simulink model "three"  (R2014b)
settings: Solver=ode23tb  StartTime=0.0  StopTime=0.1  MaxStep=.0001  MinStep=0.00001  RelTol=1e-3
libraries: powerlib x120, simulink x60, powerlib_meascontrol x1
(part 1 of 2)
settings Model: Creator=Muruganandham  LastModifiedBy=SELVA
settings DataIOCC: SignalLoggingSaveFormat=ModelDataLogs
settings OptimizationCC: ExpressionDepthLimit=2147483647
settings DebuggingCC: UnderspecifiedInitializationDetection=Classic  MergeDetectMultiDrivingBlocksExec=none  FcnCallInpInsideContextMsg=UseLocalSettings  StateNameClashWarn=warning
settings GRTTargetCC: CombineOutputUpdateFcns=off  GRTInterface=on

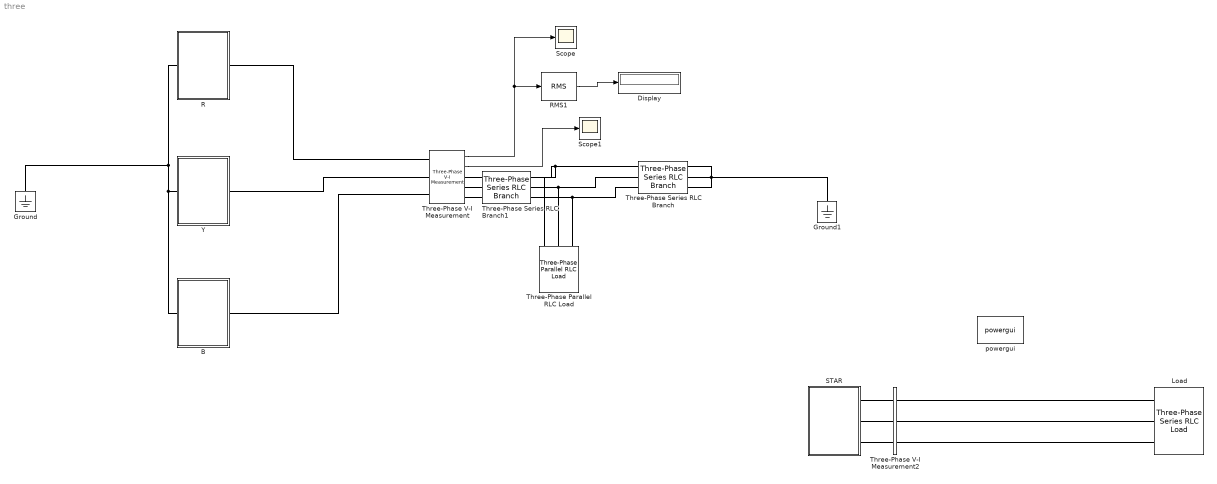
== system three ==
  " Load" : powerlib/Elements/Three-Phase Series RLC Load  LConnTagsString=A|B|C  Configuration=Delta  NominalVoltage=385  NominalFrequency=50  ActivePower=1000  InductivePower=0  CapacitivePower=0  Measurements=None  LoadType=constant Z
  "B " : Subsystem
  Display : Display
  Ground : powerlib/Elements/Ground  LConnTagsString=a
  Ground1 : powerlib/Elements/Ground  LConnTagsString=a
  R : Subsystem
  RMS1 : powerlib_meascontrol/Measurements/RMS  TrueRMS=on  Freq=50  RMSInit=00  Ts=0
  STAR : Subsystem
  Scope : Scope
      settings: YMin=-600  YMax=600  SaveName=bn  DataFormat=Structure
  Scope1 : Scope
      settings: YMin=-500  YMax=500  SaveName=ScopeData2
  Three-Phase Parallel RLC Load : powerlib/Elements/Three-Phase Parallel RLC Load  LConnTagsString=A|B|C  Configuration=Y (grounded)  NominalVoltage=380  NominalFrequency=50  ActivePower=00  InductivePower=000  CapacitivePower=3000  Measurements=None  LoadType=constant Z
  Three-Phase Series RLC Branch : powerlib/Elements/Three-Phase Series RLC Branch  LConnTagsString=A|B|C  RConnTagsString=A|B|C  BranchType=R  Resistance=10  Inductance=1e-3  Capacitance=1e-6  Measurements=None
  Three-Phase Series RLC Branch1 : powerlib/Elements/Three-Phase Series RLC Branch  LConnTagsString=A|B|C  RConnTagsString=A|B|C  BranchType=L  Resistance=10  Inductance=2e-3  Capacitance=1e-6  Measurements=None
  Three-Phase V-I Measurement : powerlib/Measurements/Three-Phase V-I Measurement  VoltageMeasurement=phase-to-phase  SetLabelV=off  LabelV=Vabc  Vpu=off  VpuLL=off  CurrentMeasurement=yes  SetLabelI=off  LabelI=Iabc  Ipu=off  Pbase=100e6  Vbase=500e3  OutputType=Complex  PhasorSimulation=off  PSBequivalent=0
  Three-Phase V-I Measurement2 : powerlib/Measurements/Three-Phase V-I Measurement  VoltageMeasurement=phase-to-phase  SetLabelV=on  LabelV=Vabc1  Vpu=off  VpuLL=off  CurrentMeasurement=yes  SetLabelI=on  LabelI=Iabc1  Ipu=off  Pbase=100e6  Vbase=500e3  OutputType=Complex  PhasorSimulation=off  PSBequivalent=0
  Y : Subsystem
  powergui : powerlib/powergui  Priority=1  SimulationMode=Discrete  SolverType=Tustin  SampleTime=50e-6  frequency=60  SPID=off  DisableSnubberDevices=off  DisableRonSwitches=off  DisableVfSwitches=off  SwTol=0  DisplayEquations=off  Interpol=off  methode=off  Ts=0  frequencyindice=0  Pbase=100e6  ErrMax=1e-4  Iterations=50  UnitsV=kV  UnitsW=MW  FunctionMessages=off  echomessages=off  HookPort=off  EnableUseOfTLC=off  x0status=blocks  RestoreLinks=warning  ResistiveCurrentMeasurement=off  Frange=[0:2:500]  Ylog=off  Xlog=on  ShowGrid=off  save=off  variable=ZData  structure=bn  ZoomFFT=off  StartTime=0.04  cycles=1  DisplayStyle=1  fundamental=50  FreqAxis=off  MaxFrequency=1000  frequencyindicesteady=1  RmsSteady=1  display=off
  wires:
  Three-Phase V-I Measurement/1 -> RMS1/1, Scope/1
  Three-Phase V-I Measurement/2 -> Scope1/1
  RMS1/1 -> Display/1
  connections:
  R/LConn1 -- Ground/LConn1 -- Y/LConn1 -- "B "/LConn1
  Three-Phase V-I Measurement/LConn1 -- R/RConn1
  Three-Phase V-I Measurement/LConn2 -- Y/RConn1
  Three-Phase V-I Measurement/LConn3 -- "B "/RConn1
  Three-Phase Series RLC Branch/LConn1 -- Three-Phase Series RLC Branch1/RConn1 -- Three-Phase Parallel RLC Load/LConn1
  Three-Phase Parallel RLC Load/LConn2 -- Three-Phase Series RLC Branch/LConn2 -- Three-Phase Series RLC Branch1/RConn2
  Three-Phase Series RLC Branch/LConn3 -- Three-Phase Parallel RLC Load/LConn3 -- Three-Phase Series RLC Branch1/RConn3
  Ground1/LConn1 -- Three-Phase Series RLC Branch/RConn3 -- Three-Phase Series RLC Branch/RConn1 -- Three-Phase Series RLC Branch/RConn2
  Three-Phase Series RLC Branch1/LConn1 -- Three-Phase V-I Measurement/RConn1
  Three-Phase V-I Measurement/RConn2 -- Three-Phase Series RLC Branch1/LConn2
  Three-Phase Series RLC Branch1/LConn3 -- Three-Phase V-I Measurement/RConn3
  STAR/LConn3 -- Three-Phase V-I Measurement2/LConn3
  Three-Phase V-I Measurement2/RConn2 -- " Load"/LConn2
  " Load"/LConn3 -- Three-Phase V-I Measurement2/RConn3
  Three-Phase V-I Measurement2/LConn2 -- STAR/LConn2
  Three-Phase V-I Measurement2/LConn1 -- STAR/LConn1
  Three-Phase V-I Measurement2/RConn1 -- " Load"/LConn1

== system three/B  ==
  B : Subsystem  mask{fc=10000, m=1}
      mask prompts: fc "Switching frequency"; m "modulation index"
  DC Voltage Source{1..3,5..6} (5 alike) : powerlib/Electrical Sources/DC Voltage Source  Amplitude=66.5  Measurements=None
  IGBT/Diode{,1..8,10..12} (12 alike) : powerlib/Power Electronics/IGBT//Diode  Ron=1e-3  Rs=1e5  Cs=inf  Measurements=on
  Scope : Scope
  Voltage Measurement : powerlib/Measurements/Voltage Measurement  PhasorSimulation=off  OutputType=Complex  PSBequivalent=0
  P : PMIOPort  Tag=PMCPort  Port=1  Side=Right
  N : PMIOPort  Tag=PMCPort  Port=2  Side=Left
  wires:
  [BS10] -> IGBT/Diode4/1
  [BS2] -> IGBT/Diode2/1
  [BS20] -> IGBT/Diode5/1
  [BS3] -> IGBT/Diode/1
  [BS30] -> IGBT/Diode3/1
  [BS40] -> IGBT/Diode8/1
  [BS6] -> IGBT/Diode6/1
  [BS4] -> IGBT/Diode12/1
  [BS5] -> IGBT/Diode7/1
  [BS50] -> IGBT/Diode10/1
  [BS60] -> IGBT/Diode11/1
  Voltage Measurement/1 -> Scope/1
  [BS1] -> IGBT/Diode1/1
  connections:
  IGBT/Diode2/RConn1 -- DC Voltage Source2/LConn1 -- IGBT/Diode/RConn1
  IGBT/Diode1/LConn1 -- DC Voltage Source1/RConn1 -- IGBT/Diode2/LConn1
  IGBT/Diode5/LConn1 -- DC Voltage Source2/RConn1 -- IGBT/Diode3/LConn1
  IGBT/Diode4/RConn1 -- DC Voltage Source1/LConn1 -- IGBT/Diode5/RConn1
  IGBT/Diode4/LConn1 -- IGBT/Diode1/RConn1 -- N/RConn1 -- Voltage Measurement/LConn2
  IGBT/Diode7/LConn1 -- DC Voltage Source6/RConn1 -- IGBT/Diode6/LConn1
  IGBT/Diode12/RConn1 -- DC Voltage Source3/LConn1 -- IGBT/Diode7/RConn1
  IGBT/Diode10/RConn1 -- DC Voltage Source6/LConn1 -- IGBT/Diode11/RConn1
  IGBT/Diode8/LConn1 -- DC Voltage Source3/RConn1 -- IGBT/Diode10/LConn1
  DC Voltage Source5/RConn1 -- IGBT/Diode/LConn1 -- IGBT/Diode12/LConn1
  DC Voltage Source5/LConn1 -- IGBT/Diode3/RConn1 -- IGBT/Diode8/RConn1
  IGBT/Diode6/RConn1 -- IGBT/Diode11/LConn1 -- P/RConn1 -- Voltage Measurement/LConn1

== system three/R ==
  DC Voltage Source{1..3,5..6} (5 alike) : powerlib/Electrical Sources/DC Voltage Source  Amplitude=66.5  Measurements=None
  IGBT/Diode{,1..8,10..12} (12 alike) : powerlib/Power Electronics/IGBT//Diode  Ron=1e-3  Rs=1e5  Cs=inf  Measurements=on
  R : Subsystem  mask{fc=10000, m=1}
      mask prompts: fc "Switching frequency"; m "modulation index"
  Scope : Scope
  Voltage Measurement : powerlib/Measurements/Voltage Measurement  PhasorSimulation=off  OutputType=Complex  PSBequivalent=0
  P : PMIOPort  Tag=PMCPort  Port=1  Side=Right
  N : PMIOPort  Tag=PMCPort  Port=2  Side=Left
  wires:
  [RS10] -> IGBT/Diode4/1
  [RS2] -> IGBT/Diode2/1
  [RS20] -> IGBT/Diode5/1
  [RS3] -> IGBT/Diode/1
  [RS30] -> IGBT/Diode3/1
  [RS40] -> IGBT/Diode8/1
  [RS6] -> IGBT/Diode6/1
  [RS4] -> IGBT/Diode12/1
  [RS5] -> IGBT/Diode7/1
  [RS50] -> IGBT/Diode10/1
  [RS60] -> IGBT/Diode11/1
  Voltage Measurement/1 -> Scope/1
  [RS1] -> IGBT/Diode1/1
  connections:
  IGBT/Diode2/RConn1 -- DC Voltage Source2/LConn1 -- IGBT/Diode/RConn1
  IGBT/Diode1/LConn1 -- DC Voltage Source1/RConn1 -- IGBT/Diode2/LConn1
  IGBT/Diode5/LConn1 -- DC Voltage Source2/RConn1 -- IGBT/Diode3/LConn1
  IGBT/Diode4/RConn1 -- DC Voltage Source1/LConn1 -- IGBT/Diode5/RConn1
  IGBT/Diode4/LConn1 -- Voltage Measurement/LConn2 -- N/RConn1 -- IGBT/Diode1/RConn1
  IGBT/Diode7/LConn1 -- DC Voltage Source6/RConn1 -- IGBT/Diode6/LConn1
  IGBT/Diode12/RConn1 -- DC Voltage Source3/LConn1 -- IGBT/Diode7/RConn1
  IGBT/Diode10/RConn1 -- DC Voltage Source6/LConn1 -- IGBT/Diode11/RConn1
  IGBT/Diode8/LConn1 -- DC Voltage Source3/RConn1 -- IGBT/Diode10/LConn1
  DC Voltage Source5/RConn1 -- IGBT/Diode/LConn1 -- IGBT/Diode12/LConn1
  DC Voltage Source5/LConn1 -- IGBT/Diode3/RConn1 -- IGBT/Diode8/RConn1
  IGBT/Diode6/RConn1 -- Voltage Measurement/LConn1 -- P/RConn1 -- IGBT/Diode11/LConn1

== system three/STAR ==
  "B " : Subsystem
  Mux : Mux  Inputs=3
  R : Subsystem
  Scope{1..3,5} (4 alike) : Scope
      Scope1 settings: YMin=-400  YMax=400  SaveName=ScopeData3
      Scope2 settings: YMin=-400  YMax=400  SaveName=ScopeData4
      Scope3 settings: YMin=-400  YMax=400  SaveName=ScopeData6
      Scope5 settings: YMin=-400  YMax=400  SaveName=bn
  Voltage Measurement1 : powerlib/Measurements/Voltage Measurement  PhasorSimulation=off  OutputType=Complex  PSBequivalent=0
  Voltage Measurement2 : powerlib/Measurements/Voltage Measurement  PhasorSimulation=off  OutputType=Complex  PSBequivalent=0
  Voltage Measurement6 : powerlib/Measurements/Voltage Measurement  PhasorSimulation=off  OutputType=Complex  PSBequivalent=0
  Y : Subsystem
  A : PMIOPort  Tag=PMCPort  Port=1  Side=Left
  B : PMIOPort  Tag=PMCPort  Port=2  Side=Left
  C : PMIOPort  Tag=PMCPort  Port=3  Side=Left
  wires:
  Voltage Measurement2/1 -> Mux/3, Scope2/1
  Voltage Measurement1/1 -> Scope1/1, Mux/2
  Voltage Measurement6/1 -> Mux/1, Scope5/1
  Mux/1 -> Scope3/1
  connections:
  Voltage Measurement6/LConn1 -- R/RConn1 -- Voltage Measurement2/LConn2 -- "B "/LConn1 -- A/RConn1
  Voltage Measurement6/LConn2 -- Voltage Measurement1/LConn1 -- R/LConn1 -- Y/RConn1 -- B/RConn1
  "B "/RConn1 -- Voltage Measurement1/LConn2 -- Y/LConn1 -- Voltage Measurement2/LConn1 -- C/RConn1

== system three/Y ==
  DC Voltage Source{1..3,5..6} (5 alike) : powerlib/Electrical Sources/DC Voltage Source  Amplitude=66.5  Measurements=None
  IGBT/Diode{,1..8,10..12} (12 alike) : powerlib/Power Electronics/IGBT//Diode  Ron=1e-3  Rs=1e5  Cs=inf  Measurements=on
  Scope : Scope
  Voltage Measurement : powerlib/Measurements/Voltage Measurement  PhasorSimulation=off  OutputType=Complex  PSBequivalent=0
  Y : Subsystem  mask{fc=10000, m=1}
      mask prompts: fc "Switching frequency"; m "modulation index"
  P : PMIOPort  Tag=PMCPort  Port=1  Side=Right
  N : PMIOPort  Tag=PMCPort  Port=2  Side=Left
  wires:
  [YS1] -> IGBT/Diode1/1
  Voltage Measurement/1 -> Scope/1
  [YS60] -> IGBT/Diode11/1
  [YS50] -> IGBT/Diode10/1
  [YS5] -> IGBT/Diode7/1
  [YS4] -> IGBT/Diode12/1
  [YS6] -> IGBT/Diode6/1
  [YS40] -> IGBT/Diode8/1
  [YS30] -> IGBT/Diode3/1
  [YS3] -> IGBT/Diode/1
  [YS20] -> IGBT/Diode5/1
  [YS2] -> IGBT/Diode2/1
  [YS10] -> IGBT/Diode4/1
  connections:
  Voltage Measurement/LConn1 -- P/RConn1 -- IGBT/Diode11/LConn1 -- IGBT/Diode6/RConn1
  IGBT/Diode8/RConn1 -- IGBT/Diode3/RConn1 -- DC Voltage Source5/LConn1
  IGBT/Diode12/LConn1 -- IGBT/Diode/LConn1 -- DC Voltage Source5/RConn1
  IGBT/Diode10/LConn1 -- IGBT/Diode8/LConn1 -- DC Voltage Source3/RConn1
  IGBT/Diode11/RConn1 -- DC Voltage Source6/LConn1 -- IGBT/Diode10/RConn1
  IGBT/Diode7/RConn1 -- IGBT/Diode12/RConn1 -- DC Voltage Source3/LConn1
  IGBT/Diode6/LConn1 -- DC Voltage Source6/RConn1 -- IGBT/Diode7/LConn1
  Voltage Measurement/LConn2 -- N/RConn1 -- IGBT/Diode1/RConn1 -- IGBT/Diode4/LConn1
  IGBT/Diode5/RConn1 -- DC Voltage Source1/LConn1 -- IGBT/Diode4/RConn1
  IGBT/Diode3/LConn1 -- DC Voltage Source2/RConn1 -- IGBT/Diode5/LConn1
  IGBT/Diode2/LConn1 -- DC Voltage Source1/RConn1 -- IGBT/Diode1/LConn1
  IGBT/Diode/RConn1 -- DC Voltage Source2/LConn1 -- IGBT/Diode2/RConn1

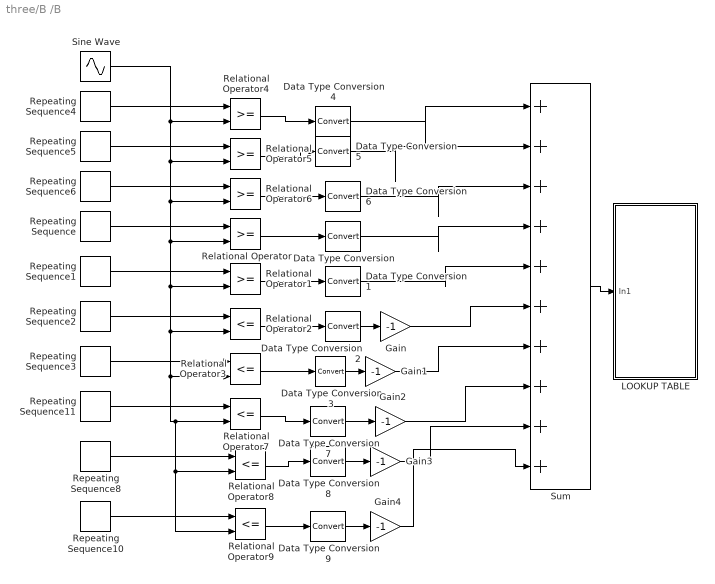
== system three/B /B ==
  Data Type Conversion{,1..9} (10 alike) : DataTypeConversion
  Gain{,1..4} (5 alike) : Gain  Gain=-1
  LOOKUP TABLE : Subsystem
  Relational Operator{,1,4..6} (5 alike) : RelationalOperator  OutDataTypeStr=boolean
  Relational Operator{2..3,7..9} (5 alike) : RelationalOperator  Operator=<=  OutDataTypeStr=boolean
  Repeating Sequence : simulink/Sources/Repeating Sequence  rep_seq_t="[0 (1/fc)/2  (1/fc)]"  rep_seq_y=[2 1 2]
  Repeating Sequence1 : simulink/Sources/Repeating Sequence  rep_seq_t="[0 (1/fc)/2  (1/fc)]"  rep_seq_y=[1 0 1]
  Repeating Sequence10 : simulink/Sources/Repeating Sequence  rep_seq_t="[0 (1/fc)/2  (1/fc)]"  rep_seq_y=[-5 -4 -5]
  Repeating Sequence11 : simulink/Sources/Repeating Sequence  rep_seq_t="[0 (1/fc)/2  (1/fc)]"  rep_seq_y=[-3 -2 -3]
  Repeating Sequence2 : simulink/Sources/Repeating Sequence  rep_seq_t="[0 (1/fc)/2  (1/fc)]"  rep_seq_y=[-1 0 -1]
  Repeating Sequence3 : simulink/Sources/Repeating Sequence  rep_seq_t="[0 (1/fc)/2  (1/fc)]"  rep_seq_y=[-2 -1 -2]
  Repeating Sequence4 : simulink/Sources/Repeating Sequence  rep_seq_t="[0 (1/fc)/2  (1/fc)]"  rep_seq_y=[4 5 4]
  Repeating Sequence5 : simulink/Sources/Repeating Sequence  rep_seq_t="[0 (1/fc)/2  (1/fc)]"  rep_seq_y=[4 3 4]
  Repeating Sequence6 : simulink/Sources/Repeating Sequence  rep_seq_t="[0 (1/fc)/2  (1/fc)]"  rep_seq_y=[3 2 3]
  Repeating Sequence8 : simulink/Sources/Repeating Sequence  rep_seq_t="[0 (1/fc)/2  (1/fc)]"  rep_seq_y=[-4 -3 -4]
  Sine Wave : Sin  Amplitude=5*m  Frequency=2*pi*50  Phase=-2*pi/3  SampleTime=0
  Sum : Sum  Inputs=|++++++++++
  wires:
  Data Type Conversion3/1 -> Gain1/1
  Data Type Conversion2/1 -> Gain/1
  Relational Operator3/1 -> Data Type Conversion3/1
  Relational Operator2/1 -> Data Type Conversion2/1
  Repeating Sequence3/1 -> Relational Operator3/1
  Repeating Sequence2/1 -> Relational Operator2/1
  Repeating Sequence1/1 -> Relational Operator1/1
  Repeating Sequence/1 -> Relational Operator/1
  Relational Operator1/1 -> Data Type Conversion1/1
  Relational Operator/1 -> Data Type Conversion/1
  Repeating Sequence6/1 -> Relational Operator6/1
  Repeating Sequence5/1 -> Relational Operator5/1
  Repeating Sequence4/1 -> Relational Operator4/1
  Relational Operator6/1 -> Data Type Conversion6/1
  Relational Operator5/1 -> Data Type Conversion5/1
  Relational Operator4/1 -> Data Type Conversion4/1
  Repeating Sequence8/1 -> Relational Operator8/1
  Repeating Sequence11/1 -> Relational Operator7/1
  Relational Operator9/1 -> Data Type Conversion9/1
  Relational Operator8/1 -> Data Type Conversion8/1
  Relational Operator7/1 -> Data Type Conversion7/1
  Data Type Conversion9/1 -> Gain4/1
  Data Type Conversion8/1 -> Gain3/1
  Data Type Conversion7/1 -> Gain2/1
  Repeating Sequence10/1 -> Relational Operator9/1
  Data Type Conversion4/1 -> Sum/1
  Data Type Conversion5/1 -> Sum/2
  Data Type Conversion6/1 -> Sum/3
  Data Type Conversion/1 -> Sum/4
  Data Type Conversion1/1 -> Sum/5
  Gain/1 -> Sum/6
  Gain1/1 -> Sum/7
  Gain2/1 -> Sum/8
  Gain3/1 -> Sum/9
  Gain4/1 -> Sum/10
  Sum/1 -> LOOKUP TABLE/1(In1)
  Sine Wave/1 -> Relational Operator5/2, Relational Operator6/2, Relational Operator/2, Relational Operator1/2, Relational Operator2/2, Relational Operator3/2, Relational Operator7/2, Relational Operator9/2, Relational Operator8/2, Relational Operator4/2

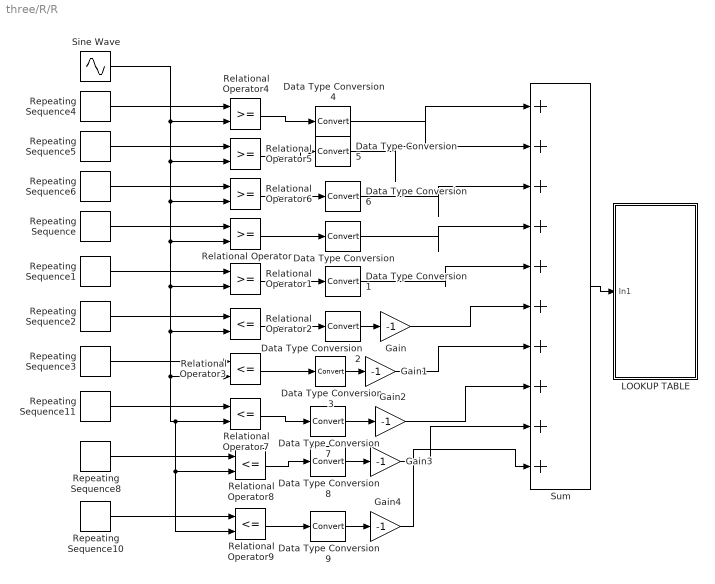
== system three/R/R ==
  Data Type Conversion{,1..9} (10 alike) : DataTypeConversion
  Gain{,1..4} (5 alike) : Gain  Gain=-1
  LOOKUP TABLE : Subsystem
  Relational Operator{,1,4..6} (5 alike) : RelationalOperator  OutDataTypeStr=boolean
  Relational Operator{2..3,7..9} (5 alike) : RelationalOperator  Operator=<=  OutDataTypeStr=boolean
  Repeating Sequence : simulink/Sources/Repeating Sequence  rep_seq_t="[0 (1/fc)/2  (1/fc)]"  rep_seq_y=[2 1 2]
  Repeating Sequence1 : simulink/Sources/Repeating Sequence  rep_seq_t="[0 (1/fc)/2  (1/fc)]"  rep_seq_y=[1 0 1]
  Repeating Sequence10 : simulink/Sources/Repeating Sequence  rep_seq_t="[0 (1/fc)/2  (1/fc)]"  rep_seq_y=[-5 -4 -5]
  Repeating Sequence11 : simulink/Sources/Repeating Sequence  rep_seq_t="[0 (1/fc)/2  (1/fc)]"  rep_seq_y=[-3 -2 -3]
  Repeating Sequence2 : simulink/Sources/Repeating Sequence  rep_seq_t="[0 (1/fc)/2  (1/fc)]"  rep_seq_y=[-1 0 -1]
  Repeating Sequence3 : simulink/Sources/Repeating Sequence  rep_seq_t="[0 (1/fc)/2  (1/fc)]"  rep_seq_y=[-2 -1 -2]
  Repeating Sequence4 : simulink/Sources/Repeating Sequence  rep_seq_t="[0 (1/fc)/2  (1/fc)]"  rep_seq_y=[4 5 4]
  Repeating Sequence5 : simulink/Sources/Repeating Sequence  rep_seq_t="[0 (1/fc)/2  (1/fc)]"  rep_seq_y=[4 3 4]
  Repeating Sequence6 : simulink/Sources/Repeating Sequence  rep_seq_t="[0 (1/fc)/2  (1/fc)]"  rep_seq_y=[3 2 3]
  Repeating Sequence8 : simulink/Sources/Repeating Sequence  rep_seq_t="[0 (1/fc)/2  (1/fc)]"  rep_seq_y=[-4 -3 -4]
  Sine Wave : Sin  Amplitude=5*m  Frequency=2*pi*50  SampleTime=0
  Sum : Sum  Inputs=|++++++++++
  wires:
  Data Type Conversion3/1 -> Gain1/1
  Data Type Conversion2/1 -> Gain/1
  Relational Operator3/1 -> Data Type Conversion3/1
  Relational Operator2/1 -> Data Type Conversion2/1
  Repeating Sequence3/1 -> Relational Operator3/1
  Repeating Sequence2/1 -> Relational Operator2/1
  Repeating Sequence1/1 -> Relational Operator1/1
  Repeating Sequence/1 -> Relational Operator/1
  Relational Operator1/1 -> Data Type Conversion1/1
  Relational Operator/1 -> Data Type Conversion/1
  Repeating Sequence6/1 -> Relational Operator6/1
  Repeating Sequence5/1 -> Relational Operator5/1
  Repeating Sequence4/1 -> Relational Operator4/1
  Relational Operator6/1 -> Data Type Conversion6/1
  Relational Operator5/1 -> Data Type Conversion5/1
  Relational Operator4/1 -> Data Type Conversion4/1
  Repeating Sequence8/1 -> Relational Operator8/1
  Repeating Sequence11/1 -> Relational Operator7/1
  Relational Operator9/1 -> Data Type Conversion9/1
  Relational Operator8/1 -> Data Type Conversion8/1
  Relational Operator7/1 -> Data Type Conversion7/1
  Data Type Conversion9/1 -> Gain4/1
  Data Type Conversion8/1 -> Gain3/1
  Data Type Conversion7/1 -> Gain2/1
  Repeating Sequence10/1 -> Relational Operator9/1
  Data Type Conversion4/1 -> Sum/1
  Data Type Conversion5/1 -> Sum/2
  Data Type Conversion6/1 -> Sum/3
  Data Type Conversion/1 -> Sum/4
  Data Type Conversion1/1 -> Sum/5
  Gain/1 -> Sum/6
  Gain1/1 -> Sum/7
  Gain2/1 -> Sum/8
  Gain3/1 -> Sum/9
  Gain4/1 -> Sum/10
  Sum/1 -> LOOKUP TABLE/1(In1)
  Sine Wave/1 -> Relational Operator5/2, Relational Operator6/2, Relational Operator/2, Relational Operator1/2, Relational Operator2/2, Relational Operator3/2, Relational Operator7/2, Relational Operator9/2, Relational Operator8/2, Relational Operator4/2

== system three/STAR/B  ==
  B : Subsystem  mask{fc=1000, m=1}
      mask prompts: fc "Switching frequency"; m "modulation index"
  DC Voltage Source{1..3,5..6} (5 alike) : powerlib/Electrical Sources/DC Voltage Source  Amplitude=66.5  Measurements=None
  IGBT/Diode{,1..8,10..12} (12 alike) : powerlib/Power Electronics/IGBT//Diode  Ron=1e-3  Rs=1e5  Cs=inf  Measurements=on
  Scope : Scope
  Voltage Measurement : powerlib/Measurements/Voltage Measurement  PhasorSimulation=off  OutputType=Complex  PSBequivalent=0
  P : PMIOPort  Tag=PMCPort  Port=1  Side=Right
  N : PMIOPort  Tag=PMCPort  Port=2  Side=Left
  wires:
  [BS10] -> IGBT/Diode4/1
  [BS2] -> IGBT/Diode2/1
  [BS20] -> IGBT/Diode5/1
  [BS3] -> IGBT/Diode/1
  [BS30] -> IGBT/Diode3/1
  [BS40] -> IGBT/Diode8/1
  [BS6] -> IGBT/Diode6/1
  [BS4] -> IGBT/Diode12/1
  [BS5] -> IGBT/Diode7/1
  [BS50] -> IGBT/Diode10/1
  [BS60] -> IGBT/Diode11/1
  Voltage Measurement/1 -> Scope/1
  [BS1] -> IGBT/Diode1/1
  connections:
  IGBT/Diode2/RConn1 -- DC Voltage Source2/LConn1 -- IGBT/Diode/RConn1
  IGBT/Diode1/LConn1 -- DC Voltage Source1/RConn1 -- IGBT/Diode2/LConn1
  IGBT/Diode5/LConn1 -- DC Voltage Source2/RConn1 -- IGBT/Diode3/LConn1
  IGBT/Diode4/RConn1 -- DC Voltage Source1/LConn1 -- IGBT/Diode5/RConn1
  IGBT/Diode4/LConn1 -- IGBT/Diode1/RConn1 -- N/RConn1 -- Voltage Measurement/LConn2
  IGBT/Diode7/LConn1 -- DC Voltage Source6/RConn1 -- IGBT/Diode6/LConn1
  IGBT/Diode12/RConn1 -- DC Voltage Source3/LConn1 -- IGBT/Diode7/RConn1
  IGBT/Diode10/RConn1 -- DC Voltage Source6/LConn1 -- IGBT/Diode11/RConn1
  IGBT/Diode8/LConn1 -- DC Voltage Source3/RConn1 -- IGBT/Diode10/LConn1
  DC Voltage Source5/RConn1 -- IGBT/Diode/LConn1 -- IGBT/Diode12/LConn1
  DC Voltage Source5/LConn1 -- IGBT/Diode3/RConn1 -- IGBT/Diode8/RConn1
  IGBT/Diode6/RConn1 -- IGBT/Diode11/LConn1 -- P/RConn1 -- Voltage Measurement/LConn1

== system three/STAR/R ==
  DC Voltage Source{1..3,5..6} (5 alike) : powerlib/Electrical Sources/DC Voltage Source  Amplitude=66.5  Measurements=None
  IGBT/Diode{,1..8,10..12} (12 alike) : powerlib/Power Electronics/IGBT//Diode  Ron=1e-3  Rs=1e5  Cs=inf  Measurements=on
  R : Subsystem  mask{fc=1000, m=1}
      mask prompts: fc "Switching frequency"; m "modulation index"
  Scope : Scope
  Voltage Measurement : powerlib/Measurements/Voltage Measurement  PhasorSimulation=off  OutputType=Complex  PSBequivalent=0
  P : PMIOPort  Tag=PMCPort  Port=1  Side=Right
  N : PMIOPort  Tag=PMCPort  Port=2  Side=Left
  wires:
  [RS10] -> IGBT/Diode4/1
  [RS2] -> IGBT/Diode2/1
  [RS20] -> IGBT/Diode5/1
  [RS3] -> IGBT/Diode/1
  [RS30] -> IGBT/Diode3/1
  [RS40] -> IGBT/Diode8/1
  [RS6] -> IGBT/Diode6/1
  [RS4] -> IGBT/Diode12/1
  [RS5] -> IGBT/Diode7/1
  [RS50] -> IGBT/Diode10/1
  [RS60] -> IGBT/Diode11/1
  Voltage Measurement/1 -> Scope/1
  [RS1] -> IGBT/Diode1/1
  connections:
  IGBT/Diode2/RConn1 -- DC Voltage Source2/LConn1 -- IGBT/Diode/RConn1
  IGBT/Diode1/LConn1 -- DC Voltage Source1/RConn1 -- IGBT/Diode2/LConn1
  IGBT/Diode5/LConn1 -- DC Voltage Source2/RConn1 -- IGBT/Diode3/LConn1
  IGBT/Diode4/RConn1 -- DC Voltage Source1/LConn1 -- IGBT/Diode5/RConn1
  IGBT/Diode4/LConn1 -- Voltage Measurement/LConn2 -- N/RConn1 -- IGBT/Diode1/RConn1
  IGBT/Diode7/LConn1 -- DC Voltage Source6/RConn1 -- IGBT/Diode6/LConn1
  IGBT/Diode12/RConn1 -- DC Voltage Source3/LConn1 -- IGBT/Diode7/RConn1
  IGBT/Diode10/RConn1 -- DC Voltage Source6/LConn1 -- IGBT/Diode11/RConn1
  IGBT/Diode8/LConn1 -- DC Voltage Source3/RConn1 -- IGBT/Diode10/LConn1
  DC Voltage Source5/RConn1 -- IGBT/Diode/LConn1 -- IGBT/Diode12/LConn1
  DC Voltage Source5/LConn1 -- IGBT/Diode3/RConn1 -- IGBT/Diode8/RConn1
  IGBT/Diode6/RConn1 -- Voltage Measurement/LConn1 -- P/RConn1 -- IGBT/Diode11/LConn1

== system three/STAR/Y ==
  B : Subsystem  mask{fc=1000, m=1}
      mask prompts: fc "Switching frequency"; m "modulation index"
  DC Voltage Source{1..3,5..6} (5 alike) : powerlib/Electrical Sources/DC Voltage Source  Amplitude=66.5  Measurements=None
  IGBT/Diode{,1..8,10..12} (12 alike) : powerlib/Power Electronics/IGBT//Diode  Ron=1e-3  Rs=1e5  Cs=inf  Measurements=on
  Scope : Scope
  Voltage Measurement : powerlib/Measurements/Voltage Measurement  PhasorSimulation=off  OutputType=Complex  PSBequivalent=0
  P : PMIOPort  Tag=PMCPort  Port=1  Side=Right
  N : PMIOPort  Tag=PMCPort  Port=2  Side=Left
  wires:
  [YS1] -> IGBT/Diode1/1
  Voltage Measurement/1 -> Scope/1
  [YS60] -> IGBT/Diode11/1
  [YS50] -> IGBT/Diode10/1
  [YS5] -> IGBT/Diode7/1
  [YS4] -> IGBT/Diode12/1
  [YS6] -> IGBT/Diode6/1
  [YS40] -> IGBT/Diode8/1
  [YS30] -> IGBT/Diode3/1
  [YS3] -> IGBT/Diode/1
  [YS20] -> IGBT/Diode5/1
  [YS2] -> IGBT/Diode2/1
  [YS10] -> IGBT/Diode4/1
  connections:
  Voltage Measurement/LConn1 -- P/RConn1 -- IGBT/Diode11/LConn1 -- IGBT/Diode6/RConn1
  IGBT/Diode8/RConn1 -- IGBT/Diode3/RConn1 -- DC Voltage Source5/LConn1
  IGBT/Diode12/LConn1 -- DC Voltage Source5/RConn1 -- IGBT/Diode/LConn1
  IGBT/Diode10/LConn1 -- DC Voltage Source3/RConn1 -- IGBT/Diode8/LConn1
  IGBT/Diode11/RConn1 -- DC Voltage Source6/LConn1 -- IGBT/Diode10/RConn1
  IGBT/Diode7/RConn1 -- DC Voltage Source3/LConn1 -- IGBT/Diode12/RConn1
  IGBT/Diode6/LConn1 -- DC Voltage Source6/RConn1 -- IGBT/Diode7/LConn1
  Voltage Measurement/LConn2 -- N/RConn1 -- IGBT/Diode1/RConn1 -- IGBT/Diode4/LConn1
  IGBT/Diode5/RConn1 -- DC Voltage Source1/LConn1 -- IGBT/Diode4/RConn1
  IGBT/Diode3/LConn1 -- DC Voltage Source2/RConn1 -- IGBT/Diode5/LConn1
  IGBT/Diode2/LConn1 -- DC Voltage Source1/RConn1 -- IGBT/Diode1/LConn1
  IGBT/Diode/RConn1 -- DC Voltage Source2/LConn1 -- IGBT/Diode2/RConn1

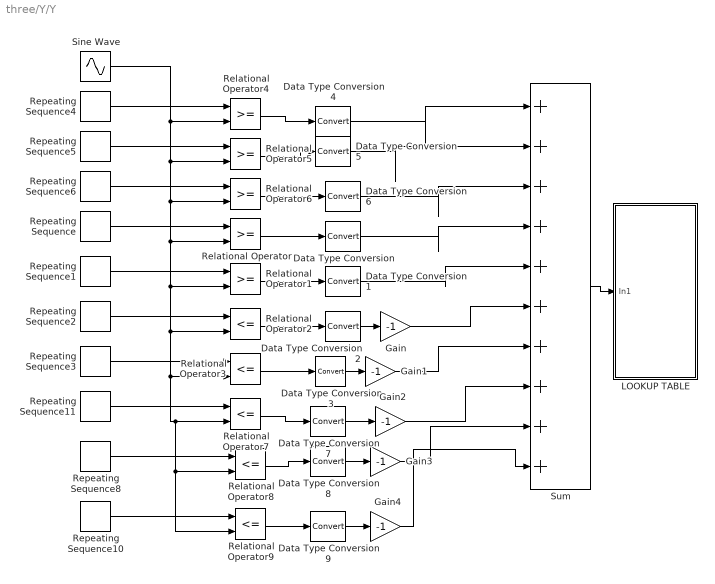
== system three/Y/Y ==
  Data Type Conversion{,1..9} (10 alike) : DataTypeConversion
  Gain{,1..4} (5 alike) : Gain  Gain=-1
  LOOKUP TABLE : Subsystem
  Relational Operator{,1,4..6} (5 alike) : RelationalOperator  OutDataTypeStr=boolean
  Relational Operator{2..3,7..9} (5 alike) : RelationalOperator  Operator=<=  OutDataTypeStr=boolean
  Repeating Sequence : simulink/Sources/Repeating Sequence  rep_seq_t="[0 (1/fc)/2  (1/fc)]"  rep_seq_y=[2 1 2]
  Repeating Sequence1 : simulink/Sources/Repeating Sequence  rep_seq_t="[0 (1/fc)/2  (1/fc)]"  rep_seq_y=[1 0 1]
  Repeating Sequence10 : simulink/Sources/Repeating Sequence  rep_seq_t="[0 (1/fc)/2  (1/fc)]"  rep_seq_y=[-5 -4 -5]
  Repeating Sequence11 : simulink/Sources/Repeating Sequence  rep_seq_t="[0 (1/fc)/2  (1/fc)]"  rep_seq_y=[-3 -2 -3]
  Repeating Sequence2 : simulink/Sources/Repeating Sequence  rep_seq_t="[0 (1/fc)/2  (1/fc)]"  rep_seq_y=[-1 0 -1]
  Repeating Sequence3 : simulink/Sources/Repeating Sequence  rep_seq_t="[0 (1/fc)/2  (1/fc)]"  rep_seq_y=[-2 -1 -2]
  Repeating Sequence4 : simulink/Sources/Repeating Sequence  rep_seq_t="[0 (1/fc)/2  (1/fc)]"  rep_seq_y=[4 5 4]
  Repeating Sequence5 : simulink/Sources/Repeating Sequence  rep_seq_t="[0 (1/fc)/2  (1/fc)]"  rep_seq_y=[4 3 4]
  Repeating Sequence6 : simulink/Sources/Repeating Sequence  rep_seq_t="[0 (1/fc)/2  (1/fc)]"  rep_seq_y=[3 2 3]
  Repeating Sequence8 : simulink/Sources/Repeating Sequence  rep_seq_t="[0 (1/fc)/2  (1/fc)]"  rep_seq_y=[-4 -3 -4]
  Sine Wave : Sin  Amplitude=5*m  Frequency=2*pi*50  Phase=2*pi/3  SampleTime=0
  Sum : Sum  Inputs=|++++++++++
  wires:
  Sine Wave/1 -> Relational Operator4/2, Relational Operator8/2, Relational Operator9/2, Relational Operator7/2, Relational Operator3/2, Relational Operator2/2, Relational Operator1/2, Relational Operator/2, Relational Operator6/2, Relational Operator5/2
  Sum/1 -> LOOKUP TABLE/1(In1)
  Gain4/1 -> Sum/10
  Gain3/1 -> Sum/9
  Gain2/1 -> Sum/8
  Gain1/1 -> Sum/7
  Gain/1 -> Sum/6
  Data Type Conversion1/1 -> Sum/5
  Data Type Conversion/1 -> Sum/4
  Data Type Conversion6/1 -> Sum/3
  Data Type Conversion5/1 -> Sum/2
  Data Type Conversion4/1 -> Sum/1
  Repeating Sequence10/1 -> Relational Operator9/1
  Data Type Conversion7/1 -> Gain2/1
  Data Type Conversion8/1 -> Gain3/1
  Data Type Conversion9/1 -> Gain4/1
  Relational Operator7/1 -> Data Type Conversion7/1
  Relational Operator8/1 -> Data Type Conversion8/1
  Relational Operator9/1 -> Data Type Conversion9/1
  Repeating Sequence11/1 -> Relational Operator7/1
  Repeating Sequence8/1 -> Relational Operator8/1
  Relational Operator4/1 -> Data Type Conversion4/1
  Relational Operator5/1 -> Data Type Conversion5/1
  Relational Operator6/1 -> Data Type Conversion6/1
  Repeating Sequence4/1 -> Relational Operator4/1
  Repeating Sequence5/1 -> Relational Operator5/1
  Repeating Sequence6/1 -> Relational Operator6/1
  Relational Operator/1 -> Data Type Conversion/1
  Relational Operator1/1 -> Data Type Conversion1/1
  Repeating Sequence/1 -> Relational Operator/1
  Repeating Sequence1/1 -> Relational Operator1/1
  Repeating Sequence2/1 -> Relational Operator2/1
  Repeating Sequence3/1 -> Relational Operator3/1
  Relational Operator2/1 -> Data Type Conversion2/1
  Relational Operator3/1 -> Data Type Conversion3/1
  Data Type Conversion2/1 -> Gain/1
  Data Type Conversion3/1 -> Gain1/1

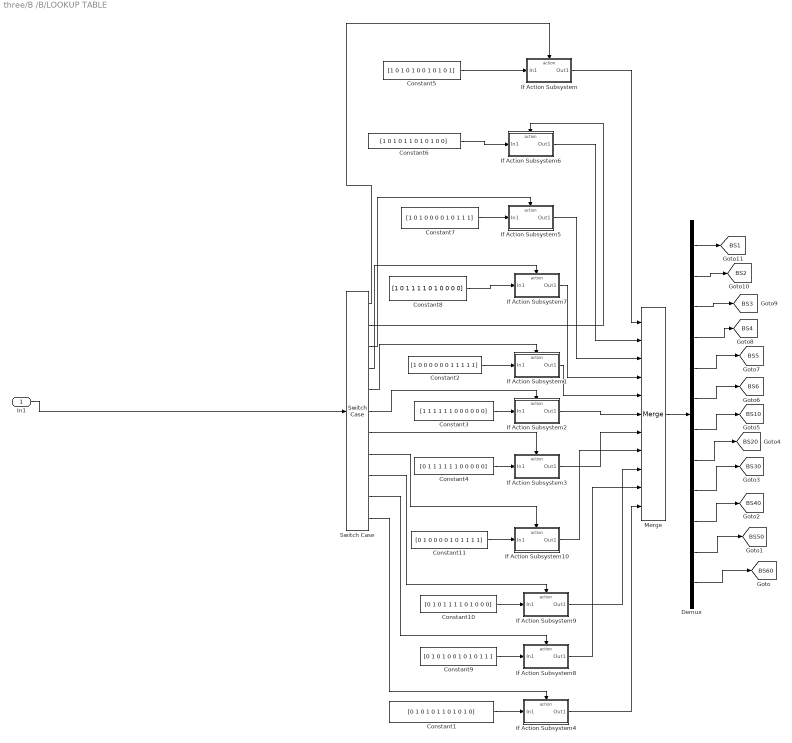
== system three/B /B/LOOKUP TABLE ==
  In1 : Inport
  Constant1 : Constant  Value=[0 1 0 1 0 1 1 0 1 0 1 0]
  Constant10 : Constant  Value=[0 1 0 1 1 1 1 0 1 0 0 0]
  Constant11 : Constant  Value=[0 1 0 0 0 0 1 0 1 1 1 1]
  Constant2 : Constant  Value=[1 0 0 0 0 0 0 1 1 1 1 1]
  Constant3 : Constant  Value=[1 1 1 1 1 1 0 0 0 0 0 0]
  Constant4 : Constant  Value=[0 1 1 1 1 1 1 0 0 0 0 0]
  Constant5 : Constant  Value=[1 0 1 0 1 0 0 1 0 1 0 1]
  Constant6 : Constant  Value=[1 0 1 0 1 1 0 1 0 1 0 0]
  Constant7 : Constant  Value=[1 0 1 0 0 0 0 1 0 1 1 1]
  Constant8 : Constant  Value=[1 0 1 1 1 1 0 1 0 0 0 0]
  Constant9 : Constant  Value=[0 1 0 1 0 0 1 0 1 0 1 1 ]
  Demux : Demux  Outputs=12
  If Action Subsystem : Subsystem  TreatAsAtomicUnit=on
  If Action Subsystem1 : Subsystem  TreatAsAtomicUnit=on
  If Action Subsystem10 : Subsystem  TreatAsAtomicUnit=on
  If Action Subsystem2 : Subsystem  TreatAsAtomicUnit=on
  If Action Subsystem3 : Subsystem  TreatAsAtomicUnit=on
  If Action Subsystem4 : Subsystem  TreatAsAtomicUnit=on
  If Action Subsystem5 : Subsystem  TreatAsAtomicUnit=on
  If Action Subsystem6 : Subsystem  TreatAsAtomicUnit=on
  If Action Subsystem7 : Subsystem  TreatAsAtomicUnit=on
  If Action Subsystem8 : Subsystem  TreatAsAtomicUnit=on
  If Action Subsystem9 : Subsystem  TreatAsAtomicUnit=on
  Merge : Merge  Inputs=11
  Switch Case : SwitchCase  CaseConditions={-5 -4 -3 -2 -1 0 1 2 3 4 5}  ShowDefaultCase=off
  tag scope: BS10=global, BS1=global, BS20=global, BS2=global, BS30=global, BS3=global, BS40=global, BS4=global, BS50=global, BS5=global, BS60=global, BS6=global
  wires:
  Merge/1 -> Demux/1
  If Action Subsystem/1(Out1) -> Merge/1
  Constant4/1 -> If Action Subsystem3/1(In1)
  Constant3/1 -> If Action Subsystem2/1(In1)
  Constant2/1 -> If Action Subsystem1/1(In1)
  Switch Case/6 -> If Action Subsystem2/Action
  If Action Subsystem6/1(Out1) -> Merge/2
  If Action Subsystem5/1(Out1) -> Merge/3
  If Action Subsystem7/1(Out1) -> Merge/4
  If Action Subsystem1/1(Out1) -> Merge/5
  If Action Subsystem2/1(Out1) -> Merge/6
  If Action Subsystem3/1(Out1) -> Merge/7
  Constant9/1 -> If Action Subsystem8/1(In1)
  Constant10/1 -> If Action Subsystem9/1(In1)
  Constant11/1 -> If Action Subsystem10/1(In1)
  Switch Case/11 -> If Action Subsystem4/Action
  If Action Subsystem4/1(Out1) -> Merge/11
  Switch Case/10 -> If Action Subsystem8/Action
  Switch Case/9 -> If Action Subsystem9/Action
  Switch Case/8 -> If Action Subsystem10/Action
  Switch Case/7 -> If Action Subsystem3/Action
  Switch Case/5 -> If Action Subsystem1/Action
  Switch Case/4 -> If Action Subsystem7/Action
  Switch Case/3 -> If Action Subsystem5/Action
  Switch Case/2 -> If Action Subsystem6/Action
  Switch Case/1 -> If Action Subsystem/Action
  Constant6/1 -> If Action Subsystem6/1(In1)
  Constant7/1 -> If Action Subsystem5/1(In1)
  Constant8/1 -> If Action Subsystem7/1(In1)
  If Action Subsystem10/1(Out1) -> Merge/8
  If Action Subsystem9/1(Out1) -> Merge/9
  If Action Subsystem8/1(Out1) -> Merge/10
  Constant1/1 -> If Action Subsystem4/1(In1)
  Constant5/1 -> If Action Subsystem/1(In1)
  In1/1 -> Switch Case/1
  Demux/1 -> [BS1]
  Demux/2 -> [BS2]
  Demux/3 -> [BS3]
  Demux/4 -> [BS4]
  Demux/6 -> [BS6]
  Demux/5 -> [BS5]
  Demux/7 -> [BS10]
  Demux/8 -> [BS20]
  Demux/11 -> [BS50]
  Demux/10 -> [BS40]
  Demux/9 -> [BS30]
  Demux/12 -> [BS60]

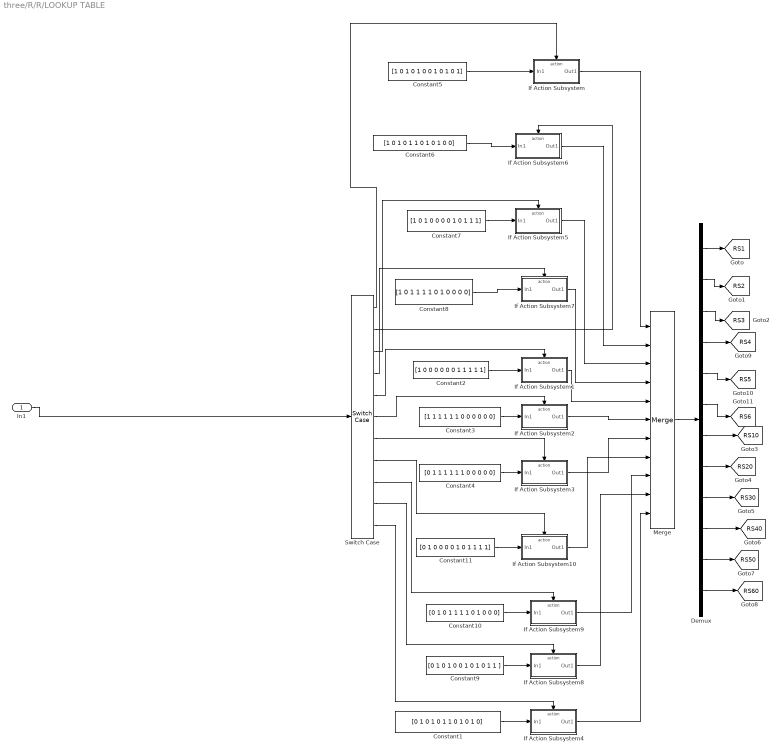
== system three/R/R/LOOKUP TABLE ==
  In1 : Inport
  Constant1 : Constant  Value=[0 1 0 1 0 1 1 0 1 0 1 0]
  Constant10 : Constant  Value=[0 1 0 1 1 1 1 0 1 0 0 0]
  Constant11 : Constant  Value=[0 1 0 0 0 0 1 0 1 1 1 1]
  Constant2 : Constant  Value=[1 0 0 0 0 0 0 1 1 1 1 1]
  Constant3 : Constant  Value=[1 1 1 1 1 1 0 0 0 0 0 0]
  Constant4 : Constant  Value=[0 1 1 1 1 1 1 0 0 0 0 0]
  Constant5 : Constant  Value=[1 0 1 0 1 0 0 1 0 1 0 1]
  Constant6 : Constant  Value=[1 0 1 0 1 1 0 1 0 1 0 0]
  Constant7 : Constant  Value=[1 0 1 0 0 0 0 1 0 1 1 1]
  Constant8 : Constant  Value=[1 0 1 1 1 1 0 1 0 0 0 0]
  Constant9 : Constant  Value=[0 1 0 1 0 0 1 0 1 0 1 1 ]
  Demux : Demux  Outputs=12
  If Action Subsystem : Subsystem  TreatAsAtomicUnit=on
  If Action Subsystem1 : Subsystem  TreatAsAtomicUnit=on
  If Action Subsystem10 : Subsystem  TreatAsAtomicUnit=on
  If Action Subsystem2 : Subsystem  TreatAsAtomicUnit=on
  If Action Subsystem3 : Subsystem  TreatAsAtomicUnit=on
  If Action Subsystem4 : Subsystem  TreatAsAtomicUnit=on
  If Action Subsystem5 : Subsystem  TreatAsAtomicUnit=on
  If Action Subsystem6 : Subsystem  TreatAsAtomicUnit=on
  If Action Subsystem7 : Subsystem  TreatAsAtomicUnit=on
  If Action Subsystem8 : Subsystem  TreatAsAtomicUnit=on
  If Action Subsystem9 : Subsystem  TreatAsAtomicUnit=on
  Merge : Merge  Inputs=11
  Switch Case : SwitchCase  CaseConditions={-5 -4 -3 -2 -1 0 1 2 3 4 5}  ShowDefaultCase=off
  tag scope: RS10=global, RS1=global, RS20=global, RS2=global, RS30=global, RS3=global, RS40=global, RS4=global, RS50=global, RS5=global, RS60=global, RS6=global
  wires:
  Merge/1 -> Demux/1
  If Action Subsystem/1(Out1) -> Merge/1
  Constant4/1 -> If Action Subsystem3/1(In1)
  Constant3/1 -> If Action Subsystem2/1(In1)
  Constant2/1 -> If Action Subsystem1/1(In1)
  Switch Case/6 -> If Action Subsystem2/Action
  If Action Subsystem6/1(Out1) -> Merge/2
  If Action Subsystem5/1(Out1) -> Merge/3
  If Action Subsystem7/1(Out1) -> Merge/4
  If Action Subsystem1/1(Out1) -> Merge/5
  If Action Subsystem2/1(Out1) -> Merge/6
  If Action Subsystem3/1(Out1) -> Merge/7
  Constant9/1 -> If Action Subsystem8/1(In1)
  Constant10/1 -> If Action Subsystem9/1(In1)
  Constant11/1 -> If Action Subsystem10/1(In1)
  Switch Case/11 -> If Action Subsystem4/Action
  If Action Subsystem4/1(Out1) -> Merge/11
  Switch Case/10 -> If Action Subsystem8/Action
  Switch Case/9 -> If Action Subsystem9/Action
  Switch Case/8 -> If Action Subsystem10/Action
  Switch Case/7 -> If Action Subsystem3/Action
  Switch Case/5 -> If Action Subsystem1/Action
  Switch Case/4 -> If Action Subsystem7/Action
  Switch Case/3 -> If Action Subsystem5/Action
  Switch Case/2 -> If Action Subsystem6/Action
  Switch Case/1 -> If Action Subsystem/Action
  Constant6/1 -> If Action Subsystem6/1(In1)
  Constant7/1 -> If Action Subsystem5/1(In1)
  Constant8/1 -> If Action Subsystem7/1(In1)
  If Action Subsystem10/1(Out1) -> Merge/8
  If Action Subsystem9/1(Out1) -> Merge/9
  If Action Subsystem8/1(Out1) -> Merge/10
  Demux/3 -> [RS3]
  Demux/2 -> [RS2]
  Demux/1 -> [RS1]
  Demux/7 -> [RS10]
  Demux/8 -> [RS20]
  Demux/9 -> [RS30]
  Demux/10 -> [RS40]
  Demux/11 -> [RS50]
  Demux/12 -> [RS60]
  Demux/6 -> [RS6]
  Demux/5 -> [RS5]
  Demux/4 -> [RS4]
  Constant1/1 -> If Action Subsystem4/1(In1)
  Constant5/1 -> If Action Subsystem/1(In1)
  In1/1 -> Switch Case/1

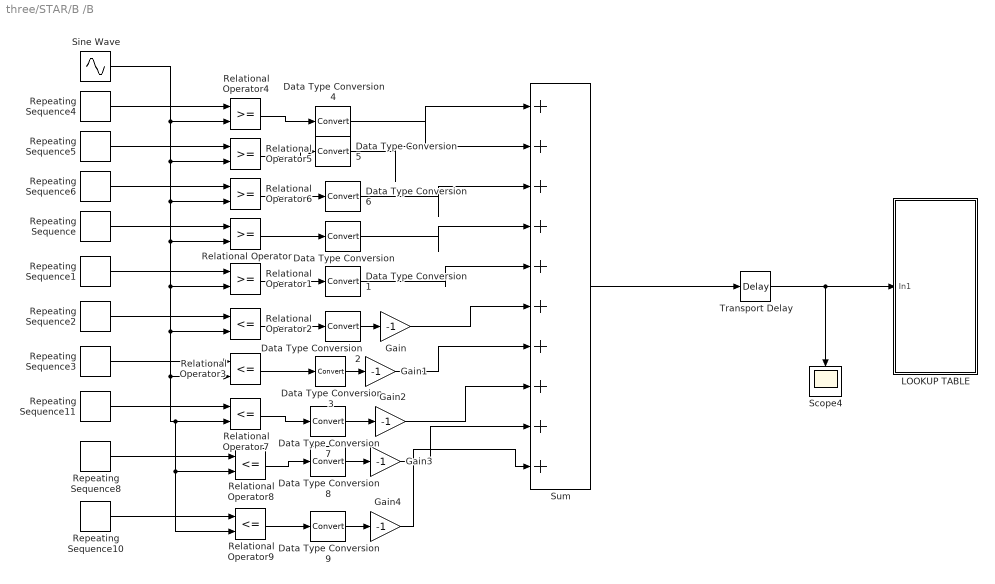
== system three/STAR/B /B ==
  Data Type Conversion{,1..9} (10 alike) : DataTypeConversion
  Gain{,1..4} (5 alike) : Gain  Gain=-1
  LOOKUP TABLE : Subsystem
  Relational Operator{,1,4..6} (5 alike) : RelationalOperator  OutDataTypeStr=boolean
  Relational Operator{2..3,7..9} (5 alike) : RelationalOperator  Operator=<=  OutDataTypeStr=boolean
  Repeating Sequence : simulink/Sources/Repeating Sequence  rep_seq_t="[0 (1/fc)/2  (1/fc)]"  rep_seq_y=[2 1 2]
  Repeating Sequence1 : simulink/Sources/Repeating Sequence  rep_seq_t="[0 (1/fc)/2  (1/fc)]"  rep_seq_y=[1 0 1]
  Repeating Sequence10 : simulink/Sources/Repeating Sequence  rep_seq_t="[0 (1/fc)/2  (1/fc)]"  rep_seq_y=[-5 -4 -5]
  Repeating Sequence11 : simulink/Sources/Repeating Sequence  rep_seq_t="[0 (1/fc)/2  (1/fc)]"  rep_seq_y=[-3 -2 -3]
  Repeating Sequence2 : simulink/Sources/Repeating Sequence  rep_seq_t="[0 (1/fc)/2  (1/fc)]"  rep_seq_y=[-1 0 -1]
  Repeating Sequence3 : simulink/Sources/Repeating Sequence  rep_seq_t="[0 (1/fc)/2  (1/fc)]"  rep_seq_y=[-2 -1 -2]
  Repeating Sequence4 : simulink/Sources/Repeating Sequence  rep_seq_t="[0 (1/fc)/2  (1/fc)]"  rep_seq_y=[4 5 4]
  Repeating Sequence5 : simulink/Sources/Repeating Sequence  rep_seq_t="[0 (1/fc)/2  (1/fc)]"  rep_seq_y=[4 3 4]
  Repeating Sequence6 : simulink/Sources/Repeating Sequence  rep_seq_t="[0 (1/fc)/2  (1/fc)]"  rep_seq_y=[3 2 3]
  Repeating Sequence8 : simulink/Sources/Repeating Sequence  rep_seq_t="[0 (1/fc)/2  (1/fc)]"  rep_seq_y=[-4 -3 -4]
  Scope4 : Scope
      settings: SaveName=ScopeData8
  Sine Wave : Sin  Amplitude=5*m  Frequency=2*pi*50  SampleTime=0
  Sum : Sum  Inputs=|++++++++++
  Transport Delay : TransportDelay  DelayTime=(0.01*7)/5
  wires:
  Data Type Conversion3/1 -> Gain1/1
  Data Type Conversion2/1 -> Gain/1
  Relational Operator3/1 -> Data Type Conversion3/1
  Relational Operator2/1 -> Data Type Conversion2/1
  Repeating Sequence3/1 -> Relational Operator3/1
  Repeating Sequence2/1 -> Relational Operator2/1
  Repeating Sequence1/1 -> Relational Operator1/1
  Repeating Sequence/1 -> Relational Operator/1
  Relational Operator1/1 -> Data Type Conversion1/1
  Relational Operator/1 -> Data Type Conversion/1
  Repeating Sequence6/1 -> Relational Operator6/1
  Repeating Sequence5/1 -> Relational Operator5/1
  Repeating Sequence4/1 -> Relational Operator4/1
  Relational Operator6/1 -> Data Type Conversion6/1
  Relational Operator5/1 -> Data Type Conversion5/1
  Relational Operator4/1 -> Data Type Conversion4/1
  Repeating Sequence8/1 -> Relational Operator8/1
  Repeating Sequence11/1 -> Relational Operator7/1
  Relational Operator9/1 -> Data Type Conversion9/1
  Relational Operator8/1 -> Data Type Conversion8/1
  Relational Operator7/1 -> Data Type Conversion7/1
  Data Type Conversion9/1 -> Gain4/1
  Data Type Conversion8/1 -> Gain3/1
  Data Type Conversion7/1 -> Gain2/1
  Repeating Sequence10/1 -> Relational Operator9/1
  Data Type Conversion4/1 -> Sum/1
  Data Type Conversion5/1 -> Sum/2
  Data Type Conversion6/1 -> Sum/3
  Data Type Conversion/1 -> Sum/4
  Data Type Conversion1/1 -> Sum/5
  Gain/1 -> Sum/6
  Gain1/1 -> Sum/7
  Gain2/1 -> Sum/8
  Gain3/1 -> Sum/9
  Gain4/1 -> Sum/10
  Sine Wave/1 -> Relational Operator5/2, Relational Operator6/2, Relational Operator/2, Relational Operator1/2, Relational Operator2/2, Relational Operator3/2, Relational Operator7/2, Relational Operator9/2, Relational Operator8/2, Relational Operator4/2
  Sum/1 -> Transport Delay/1
  Transport Delay/1 -> Scope4/1, LOOKUP TABLE/1(In1)

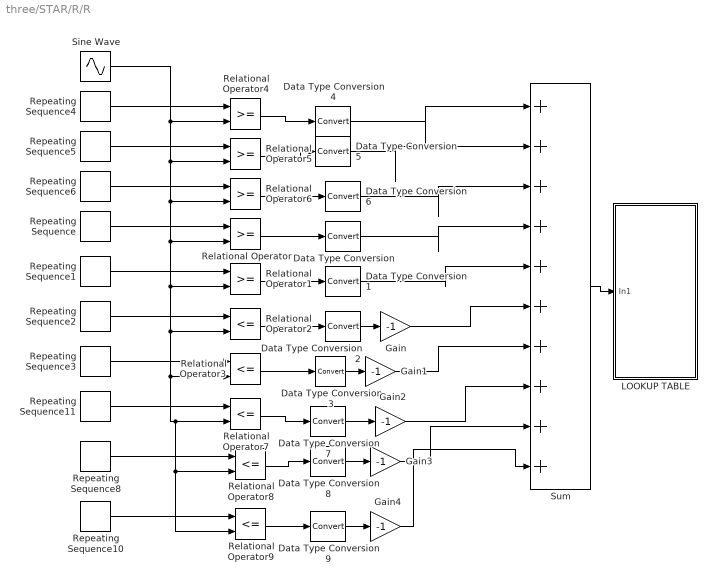
== system three/STAR/R/R ==
  Data Type Conversion{,1..9} (10 alike) : DataTypeConversion
  Gain{,1..4} (5 alike) : Gain  Gain=-1
  LOOKUP TABLE : Subsystem
  Relational Operator{,1,4..6} (5 alike) : RelationalOperator  OutDataTypeStr=boolean
  Relational Operator{2..3,7..9} (5 alike) : RelationalOperator  Operator=<=  OutDataTypeStr=boolean
  Repeating Sequence : simulink/Sources/Repeating Sequence  rep_seq_t="[0 (1/fc)/2  (1/fc)]"  rep_seq_y=[2 1 2]
  Repeating Sequence1 : simulink/Sources/Repeating Sequence  rep_seq_t="[0 (1/fc)/2  (1/fc)]"  rep_seq_y=[1 0 1]
  Repeating Sequence10 : simulink/Sources/Repeating Sequence  rep_seq_t="[0 (1/fc)/2  (1/fc)]"  rep_seq_y=[-5 -4 -5]
  Repeating Sequence11 : simulink/Sources/Repeating Sequence  rep_seq_t="[0 (1/fc)/2  (1/fc)]"  rep_seq_y=[-3 -2 -3]
  Repeating Sequence2 : simulink/Sources/Repeating Sequence  rep_seq_t="[0 (1/fc)/2  (1/fc)]"  rep_seq_y=[-1 0 -1]
  Repeating Sequence3 : simulink/Sources/Repeating Sequence  rep_seq_t="[0 (1/fc)/2  (1/fc)]"  rep_seq_y=[-2 -1 -2]
  Repeating Sequence4 : simulink/Sources/Repeating Sequence  rep_seq_t="[0 (1/fc)/2  (1/fc)]"  rep_seq_y=[4 5 4]
  Repeating Sequence5 : simulink/Sources/Repeating Sequence  rep_seq_t="[0 (1/fc)/2  (1/fc)]"  rep_seq_y=[4 3 4]
  Repeating Sequence6 : simulink/Sources/Repeating Sequence  rep_seq_t="[0 (1/fc)/2  (1/fc)]"  rep_seq_y=[3 2 3]
  Repeating Sequence8 : simulink/Sources/Repeating Sequence  rep_seq_t="[0 (1/fc)/2  (1/fc)]"  rep_seq_y=[-4 -3 -4]
  Sine Wave : Sin  Amplitude=5*m  Frequency=2*pi*50  SampleTime=0
  Sum : Sum  Inputs=|++++++++++
  wires:
  Data Type Conversion3/1 -> Gain1/1
  Data Type Conversion2/1 -> Gain/1
  Relational Operator3/1 -> Data Type Conversion3/1
  Relational Operator2/1 -> Data Type Conversion2/1
  Repeating Sequence3/1 -> Relational Operator3/1
  Repeating Sequence2/1 -> Relational Operator2/1
  Repeating Sequence1/1 -> Relational Operator1/1
  Repeating Sequence/1 -> Relational Operator/1
  Relational Operator1/1 -> Data Type Conversion1/1
  Relational Operator/1 -> Data Type Conversion/1
  Repeating Sequence6/1 -> Relational Operator6/1
  Repeating Sequence5/1 -> Relational Operator5/1
  Repeating Sequence4/1 -> Relational Operator4/1
  Relational Operator6/1 -> Data Type Conversion6/1
  Relational Operator5/1 -> Data Type Conversion5/1
  Relational Operator4/1 -> Data Type Conversion4/1
  Repeating Sequence8/1 -> Relational Operator8/1
  Repeating Sequence11/1 -> Relational Operator7/1
  Relational Operator9/1 -> Data Type Conversion9/1
  Relational Operator8/1 -> Data Type Conversion8/1
  Relational Operator7/1 -> Data Type Conversion7/1
  Data Type Conversion9/1 -> Gain4/1
  Data Type Conversion8/1 -> Gain3/1
  Data Type Conversion7/1 -> Gain2/1
  Repeating Sequence10/1 -> Relational Operator9/1
  Data Type Conversion4/1 -> Sum/1
  Data Type Conversion5/1 -> Sum/2
  Data Type Conversion6/1 -> Sum/3
  Data Type Conversion/1 -> Sum/4
  Data Type Conversion1/1 -> Sum/5
  Gain/1 -> Sum/6
  Gain1/1 -> Sum/7
  Gain2/1 -> Sum/8
  Gain3/1 -> Sum/9
  Gain4/1 -> Sum/10
  Sum/1 -> LOOKUP TABLE/1(In1)
  Sine Wave/1 -> Relational Operator5/2, Relational Operator6/2, Relational Operator/2, Relational Operator1/2, Relational Operator2/2, Relational Operator3/2, Relational Operator7/2, Relational Operator9/2, Relational Operator8/2, Relational Operator4/2

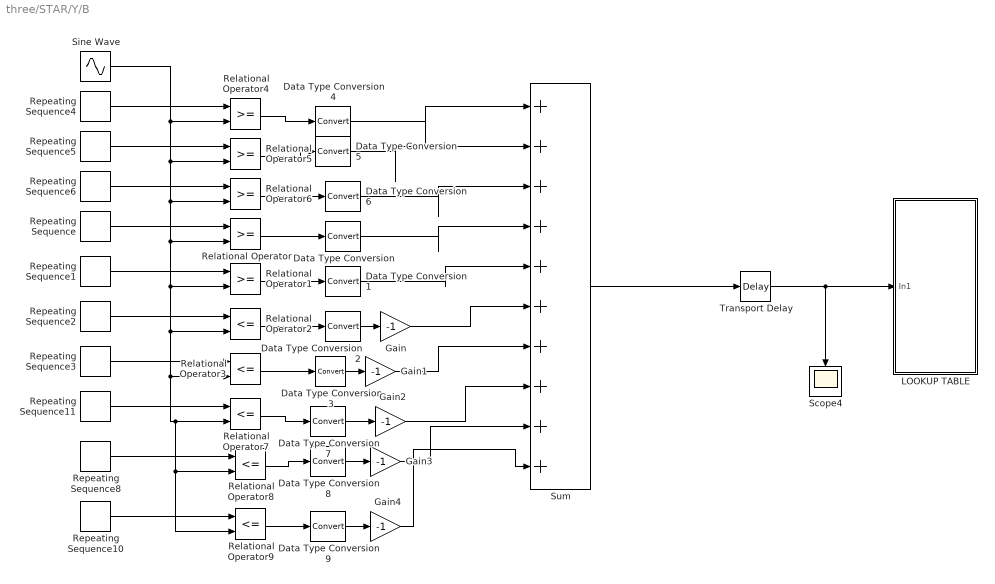
== system three/STAR/Y/B ==
  Data Type Conversion{,1..9} (10 alike) : DataTypeConversion
  Gain{,1..4} (5 alike) : Gain  Gain=-1
  LOOKUP TABLE : Subsystem
  Relational Operator{,1,4..6} (5 alike) : RelationalOperator  OutDataTypeStr=boolean
  Relational Operator{2..3,7..9} (5 alike) : RelationalOperator  Operator=<=  OutDataTypeStr=boolean
  Repeating Sequence : simulink/Sources/Repeating Sequence  rep_seq_t="[0 (1/fc)/2  (1/fc)]"  rep_seq_y=[2 1 2]
  Repeating Sequence1 : simulink/Sources/Repeating Sequence  rep_seq_t="[0 (1/fc)/2  (1/fc)]"  rep_seq_y=[1 0 1]
  Repeating Sequence10 : simulink/Sources/Repeating Sequence  rep_seq_t="[0 (1/fc)/2  (1/fc)]"  rep_seq_y=[-5 -4 -5]
  Repeating Sequence11 : simulink/Sources/Repeating Sequence  rep_seq_t="[0 (1/fc)/2  (1/fc)]"  rep_seq_y=[-3 -2 -3]
  Repeating Sequence2 : simulink/Sources/Repeating Sequence  rep_seq_t="[0 (1/fc)/2  (1/fc)]"  rep_seq_y=[-1 0 -1]
  Repeating Sequence3 : simulink/Sources/Repeating Sequence  rep_seq_t="[0 (1/fc)/2  (1/fc)]"  rep_seq_y=[-2 -1 -2]
  Repeating Sequence4 : simulink/Sources/Repeating Sequence  rep_seq_t="[0 (1/fc)/2  (1/fc)]"  rep_seq_y=[4 5 4]
  Repeating Sequence5 : simulink/Sources/Repeating Sequence  rep_seq_t="[0 (1/fc)/2  (1/fc)]"  rep_seq_y=[4 3 4]
  Repeating Sequence6 : simulink/Sources/Repeating Sequence  rep_seq_t="[0 (1/fc)/2  (1/fc)]"  rep_seq_y=[3 2 3]
  Repeating Sequence8 : simulink/Sources/Repeating Sequence  rep_seq_t="[0 (1/fc)/2  (1/fc)]"  rep_seq_y=[-4 -3 -4]
  Scope4 : Scope
      settings: SaveName=ScopeData8
  Sine Wave : Sin  Amplitude=5*m  Frequency=2*pi*50  SampleTime=0
  Sum : Sum  Inputs=|++++++++++
  Transport Delay : TransportDelay  DelayTime=(0.01*7)/10
  wires:
  Transport Delay/1 -> LOOKUP TABLE/1(In1), Scope4/1
  Sum/1 -> Transport Delay/1
  Sine Wave/1 -> Relational Operator4/2, Relational Operator8/2, Relational Operator9/2, Relational Operator7/2, Relational Operator3/2, Relational Operator2/2, Relational Operator1/2, Relational Operator/2, Relational Operator6/2, Relational Operator5/2
  Gain4/1 -> Sum/10
  Gain3/1 -> Sum/9
  Gain2/1 -> Sum/8
  Gain1/1 -> Sum/7
  Gain/1 -> Sum/6
  Data Type Conversion1/1 -> Sum/5
  Data Type Conversion/1 -> Sum/4
  Data Type Conversion6/1 -> Sum/3
  Data Type Conversion5/1 -> Sum/2
  Data Type Conversion4/1 -> Sum/1
  Repeating Sequence10/1 -> Relational Operator9/1
  Data Type Conversion7/1 -> Gain2/1
  Data Type Conversion8/1 -> Gain3/1
  Data Type Conversion9/1 -> Gain4/1
  Relational Operator7/1 -> Data Type Conversion7/1
  Relational Operator8/1 -> Data Type Conversion8/1
  Relational Operator9/1 -> Data Type Conversion9/1
  Repeating Sequence11/1 -> Relational Operator7/1
  Repeating Sequence8/1 -> Relational Operator8/1
  Relational Operator4/1 -> Data Type Conversion4/1
  Relational Operator5/1 -> Data Type Conversion5/1
  Relational Operator6/1 -> Data Type Conversion6/1
  Repeating Sequence4/1 -> Relational Operator4/1
  Repeating Sequence5/1 -> Relational Operator5/1
  Repeating Sequence6/1 -> Relational Operator6/1
  Relational Operator/1 -> Data Type Conversion/1
  Relational Operator1/1 -> Data Type Conversion1/1
  Repeating Sequence/1 -> Relational Operator/1
  Repeating Sequence1/1 -> Relational Operator1/1
  Repeating Sequence2/1 -> Relational Operator2/1
  Repeating Sequence3/1 -> Relational Operator3/1
  Relational Operator2/1 -> Data Type Conversion2/1
  Relational Operator3/1 -> Data Type Conversion3/1
  Data Type Conversion2/1 -> Gain/1
  Data Type Conversion3/1 -> Gain1/1

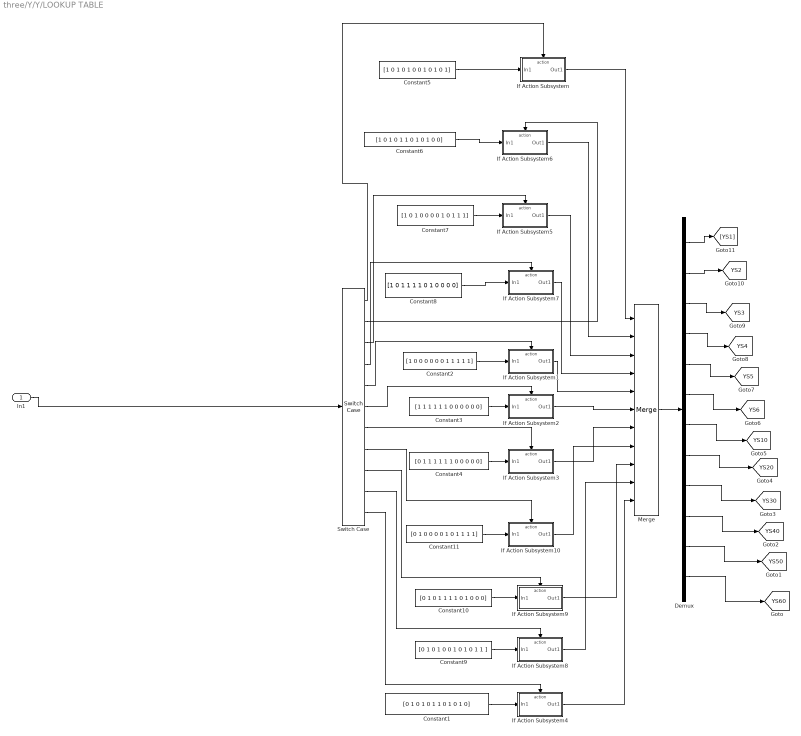
== system three/Y/Y/LOOKUP TABLE ==
  In1 : Inport
  Constant1 : Constant  Value=[0 1 0 1 0 1 1 0 1 0 1 0]
  Constant10 : Constant  Value=[0 1 0 1 1 1 1 0 1 0 0 0]
  Constant11 : Constant  Value=[0 1 0 0 0 0 1 0 1 1 1 1]
  Constant2 : Constant  Value=[1 0 0 0 0 0 0 1 1 1 1 1]
  Constant3 : Constant  Value=[1 1 1 1 1 1 0 0 0 0 0 0]
  Constant4 : Constant  Value=[0 1 1 1 1 1 1 0 0 0 0 0]
  Constant5 : Constant  Value=[1 0 1 0 1 0 0 1 0 1 0 1]
  Constant6 : Constant  Value=[1 0 1 0 1 1 0 1 0 1 0 0]
  Constant7 : Constant  Value=[1 0 1 0 0 0 0 1 0 1 1 1]
  Constant8 : Constant  Value=[1 0 1 1 1 1 0 1 0 0 0 0]
  Constant9 : Constant  Value=[0 1 0 1 0 0 1 0 1 0 1 1 ]
  Demux : Demux  Outputs=12
  If Action Subsystem : Subsystem  TreatAsAtomicUnit=on
  If Action Subsystem1 : Subsystem  TreatAsAtomicUnit=on
  If Action Subsystem10 : Subsystem  TreatAsAtomicUnit=on
  If Action Subsystem2 : Subsystem  TreatAsAtomicUnit=on
  If Action Subsystem3 : Subsystem  TreatAsAtomicUnit=on
  If Action Subsystem4 : Subsystem  TreatAsAtomicUnit=on
  If Action Subsystem5 : Subsystem  TreatAsAtomicUnit=on
  If Action Subsystem6 : Subsystem  TreatAsAtomicUnit=on
  If Action Subsystem7 : Subsystem  TreatAsAtomicUnit=on
  If Action Subsystem8 : Subsystem  TreatAsAtomicUnit=on
  If Action Subsystem9 : Subsystem  TreatAsAtomicUnit=on
  Merge : Merge  Inputs=11
  Switch Case : SwitchCase  CaseConditions={-5 -4 -3 -2 -1 0 1 2 3 4 5}  ShowDefaultCase=off
  tag scope: YS10=global, YS20=global, YS2=global, YS30=global, YS3=global, YS40=global, YS4=global, YS50=global, YS5=global, YS60=global, YS6=global
  wires:
  In1/1 -> Switch Case/1
  Constant5/1 -> If Action Subsystem/1(In1)
  Constant1/1 -> If Action Subsystem4/1(In1)
  If Action Subsystem8/1(Out1) -> Merge/10
  If Action Subsystem9/1(Out1) -> Merge/9
  If Action Subsystem10/1(Out1) -> Merge/8
  Constant8/1 -> If Action Subsystem7/1(In1)
  Constant7/1 -> If Action Subsystem5/1(In1)
  Constant6/1 -> If Action Subsystem6/1(In1)
  Switch Case/1 -> If Action Subsystem/Action
  Switch Case/2 -> If Action Subsystem6/Action
  Switch Case/3 -> If Action Subsystem5/Action
  Switch Case/4 -> If Action Subsystem7/Action
  Switch Case/5 -> If Action Subsystem1/Action
  Switch Case/7 -> If Action Subsystem3/Action
  Switch Case/8 -> If Action Subsystem10/Action
  Switch Case/9 -> If Action Subsystem9/Action
  Switch Case/10 -> If Action Subsystem8/Action
  If Action Subsystem4/1(Out1) -> Merge/11
  Switch Case/11 -> If Action Subsystem4/Action
  Constant11/1 -> If Action Subsystem10/1(In1)
  Constant10/1 -> If Action Subsystem9/1(In1)
  Constant9/1 -> If Action Subsystem8/1(In1)
  If Action Subsystem3/1(Out1) -> Merge/7
  If Action Subsystem2/1(Out1) -> Merge/6
  If Action Subsystem1/1(Out1) -> Merge/5
  If Action Subsystem7/1(Out1) -> Merge/4
  If Action Subsystem5/1(Out1) -> Merge/3
  If Action Subsystem6/1(Out1) -> Merge/2
  Switch Case/6 -> If Action Subsystem2/Action
  Constant2/1 -> If Action Subsystem1/1(In1)
  Constant3/1 -> If Action Subsystem2/1(In1)
  Constant4/1 -> If Action Subsystem3/1(In1)
  If Action Subsystem/1(Out1) -> Merge/1
  Merge/1 -> Demux/1
  Demux/1 -> [YS1]
  Demux/2 -> [YS2]
  Demux/3 -> [YS3]
  Demux/4 -> [YS4]
  Demux/5 -> [YS5]
  Demux/6 -> [YS6]
  Demux/7 -> [YS10]
  Demux/8 -> [YS20]
  Demux/9 -> [YS30]
  Demux/10 -> [YS40]
  Demux/11 -> [YS50]
  Demux/12 -> [YS60]

== system three/B /B/LOOKUP TABLE/If Action Subsystem ==
  In1 : Inport
  Action Port : ActionPort  ActionType=case
  Out1 : Outport
  wires:
  In1/1 -> Out1/1

== system three/B /B/LOOKUP TABLE/If Action Subsystem1 ==
  In1 : Inport
  Action Port : ActionPort  ActionType=case
  Out1 : Outport
  wires:
  In1/1 -> Out1/1

== system three/B /B/LOOKUP TABLE/If Action Subsystem10 ==
  In1 : Inport
  Action Port : ActionPort  ActionType=case
  Out1 : Outport
  wires:
  In1/1 -> Out1/1

== system three/B /B/LOOKUP TABLE/If Action Subsystem2 ==
  In1 : Inport
  Action Port : ActionPort  ActionType=case
  Out1 : Outport
  wires:
  In1/1 -> Out1/1

== system three/B /B/LOOKUP TABLE/If Action Subsystem3 ==
  In1 : Inport
  Action Port : ActionPort  ActionType=case
  Out1 : Outport
  wires:
  In1/1 -> Out1/1

== system three/B /B/LOOKUP TABLE/If Action Subsystem4 ==
  In1 : Inport
  Action Port : ActionPort  ActionType=case
  Out1 : Outport
  wires:
  In1/1 -> Out1/1

== system three/B /B/LOOKUP TABLE/If Action Subsystem5 ==
  In1 : Inport
  Action Port : ActionPort  ActionType=case
  Out1 : Outport
  wires:
  In1/1 -> Out1/1

== system three/B /B/LOOKUP TABLE/If Action Subsystem6 ==
  In1 : Inport
  Action Port : ActionPort  ActionType=case
  Out1 : Outport
  wires:
  In1/1 -> Out1/1

== system three/B /B/LOOKUP TABLE/If Action Subsystem7 ==
  In1 : Inport
  Action Port : ActionPort  ActionType=case
  Out1 : Outport
  wires:
  In1/1 -> Out1/1

== system three/B /B/LOOKUP TABLE/If Action Subsystem8 ==
  In1 : Inport
  Action Port : ActionPort  ActionType=case
  Out1 : Outport
  wires:
  In1/1 -> Out1/1

== system three/B /B/LOOKUP TABLE/If Action Subsystem9 ==
  In1 : Inport
  Action Port : ActionPort  ActionType=case
  Out1 : Outport
  wires:
  In1/1 -> Out1/1

== system three/R/R/LOOKUP TABLE/If Action Subsystem ==
  In1 : Inport
  Action Port : ActionPort  ActionType=case
  Out1 : Outport
  wires:
  In1/1 -> Out1/1
